simulink model "MSFartoystyring_2_CAC"  (R2018a)
settings: Solver=ode45  StartTime=tstart  StopTime=tstop  RelTol=1e-3  EnableMultiTasking=on
values from neighbouring files (symbols this model uses):
  c = 1    [run_2.m]    (also in run_task_1_4.m; run_task_1_6.m = 0; run_task_1_8_new.m)
  chi_t = atan2(WP(2,2)-WP(2,1),WP(1,2)-WP(1,1))    [run_2.m]
  dc_max = 25*(pi/180)    (= 0.436332312999)    [run_2.m]    (also in run_task_1_8_new.m)
  delta_e = 3*304.8    (= 914.4)    [run_2.m]
  delta_s = 3*304.8    (= 914.4)    [run_2.m]
  e_d = 2*304.8    (= 609.6)    [run_2.m]
  kappa = nc_max - U_t    (= 5.90117918517)    [run_2.m]
  kd_heading = 2*zeta*omegan*(m+km)-d    [run_2.m]    (also in run_task_1_8_new.m)
  kd_surge = 0    [run_2.m]
  ki_heading = omegan/10*kp_heading    [run_2.m]    (also in run_task_1_8_new.m)
  ki_surge = 0    [run_2.m]    (also in run_task_1_8_new.m = lambda^2)
  kp_heading = (m+km)*omegan^2-k    [run_2.m]    (also in run_task_1_8_new.m)
  kp_surge = 100    [run_2.m]    (also in run_task_1_8_new.m = 2*lambda)
  nc_max = (85/60)*2*pi    (= 8.90117918517)    [run_2.m]    (also in run_task_1_8_new.m)
  p0 = [1000 700]'    [run_2.m]    (also in run_task_1_4.m = zeros(2,1); run_task_1_6.m = zeros(2,1); run_task_1_8_new.m = zeros(2,1))
  psi0 = 60*pi/180    (= 1.0471975512)    [run_2.m]    (also in run_task_1_4.m = 0; run_task_1_6.m = 0; run_task_1_8_new.m = 0)
  r0 = 0    [run_2.m]    (also in run_task_1_4.m; run_task_1_6.m; run_task_1_8_new.m)
  s_d = 1*304.8    (= 304.8)    [run_2.m]
  tsamp = 10    [run_2.m]    (also in run_task_1_4.m; run_task_1_6.m; run_task_1_8_new.m)
  U_t = 3    [run_2.m]
  v0 = [6.63 0]'    [run_2.m]    (also in run_task_1_4.m; run_task_1_6.m = [0.001 0]'; run_task_1_8_new.m = [3 0]')
undefined symbols (not defined in the file or in its folder): msfartoystyring
settings Model: ExtModeAutoUpdateStatusClock=off  Creator=christh  LastModifiedBy=Anders Vagle
settings SolverCC: ZeroCrossAlgorithm=Adaptive
settings DataIOCC: LimitDataPoints=on  SaveFormat=Array
settings OptimizationCC: ExpressionDepthLimit=2147483647  InitFltsAndDblsToZero=on  LifeSpan=inf
settings DebuggingCC: UnderspecifiedInitializationDetection=Classic  MergeDetectMultiDrivingBlocksExec=none  MaxConsecutiveZCsMsg=none  SolverPrmCheckMsg=warning  FcnCallInpInsideContextMsg=warning  StateNameClashWarn=warning  SFUnexpectedBacktrackingDiag=warning  SFNoUnconditionalDefaultTransitionDiag=warning  SFExecutionAtInitializationDiag=none
settings HardwareCC: ProdBitPerPointer=32  ProdBitPerSizeT=32  ProdBitPerPtrDiffT=32  ProdLargestAtomicFloat=None  ProdIntDivRoundTo=Undefined  ProdEndianess=Unspecified  ProdWordSize=32  ProdHWDeviceType=32-bit Generic
settings ModelReferenceCC: PropagateSignalLabelsOutOfModel=off
settings CodeAppCC: StateflowObjectComments=on
settings GRTTargetCC: TargetLangStandard=C89/C90 (ANSI)  GeneratePreprocessorConditionals=Disable all  CombineOutputUpdateFcns=off  GRTInterface=on
settings ConfigComp: CovMetricSettings=dw  CovHtmlReporting=on  CovSaveCumulativeToWorkspaceVar=on  CovSaveSingleToWorkspaceVar=on  CovExternalEMLEnable=off

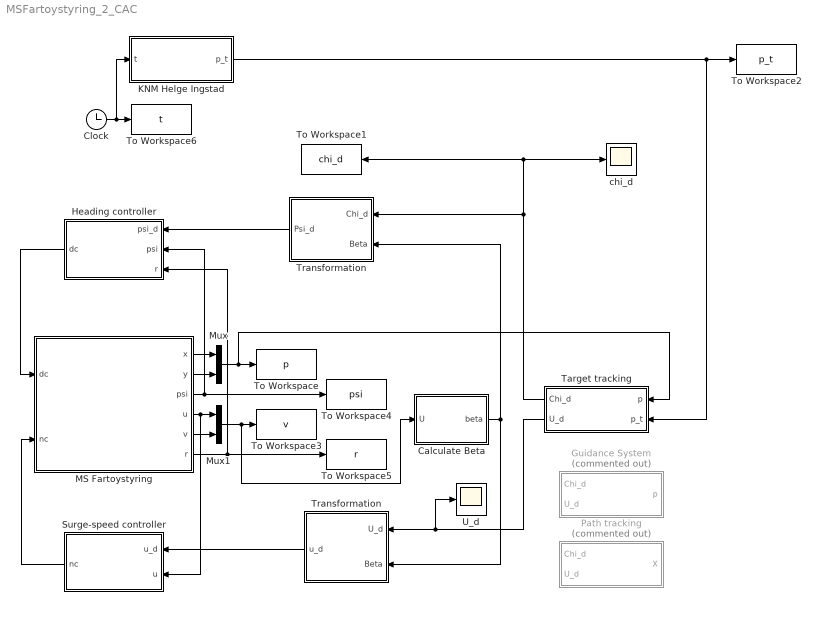
== system MSFartoystyring_2_CAC ==
  Calculate Beta : MATLAB Function  TreatAsAtomicUnit=on
  Clock : Clock
  Guidance System : Subsystem  Commented=on
  Heading controller : Subsystem
  KNM Helge Ingstad : Subsystem
  MS Fartoystyring : Subsystem  mask(MS Fartoystyring for Assignment 3 G&C){x0=p0(1), y0=p0(2), u0=v0(1), v0=v0(2), psi0=psi0, r0=r0, c=c}
      mask prompts: x0 "x(t0) (m)"; y0 "y(t0) (m)"; u0 "u(t0) (m/s)"; v0 "v(t0) (m/s)"; psi0 "psi(t0) (rad)"; r0 "r(t0) (rad/s)"; c "current (0 or 1)"
      mask help:
      | Block corresponding to Figure 1 in the assignment text. Gives the response of the ship.
      |
      | The design speed of MS Fartoystyring is u=8.23 m/s.
      |
      | Input:
      | dc: commanded rudder (rad), dmax=25*pi/180
      | nc: commanded shaft speed (rad/s), nmax=85*2*pi/60
      |
      | Output:
      | x: north pos (m)
      | y: east pos (m)
      | u: surge (m/s)
      | v: sway (m/s)
      | psi: heading (rad)
      | r: yaw (rad/s)
      mask Help: Comments, bugs and help requests can be directed to the TA. Email on course website.
  Mux : Mux  Inputs=2
  Mux1 : Mux  Inputs=2
  Path tracking : Subsystem  Commented=on
  Surge-speed controller : Subsystem
  Target tracking : Subsystem
  To Workspace : ToWorkspace  VariableName=p  SampleTime=tsamp
  To Workspace1 : ToWorkspace  VariableName=chi_d  SampleTime=tsamp
  To Workspace2 : ToWorkspace  VariableName=p_t  SampleTime=tsamp
  To Workspace3 : ToWorkspace  VariableName=v  SampleTime=tsamp
  To Workspace4 : ToWorkspace  VariableName=psi  SampleTime=tsamp
  To Workspace5 : ToWorkspace  VariableName=r  SampleTime=tsamp
  To Workspace6 : ToWorkspace  VariableName=t  SampleTime=tsamp
  Transformation : Subsystem
  "Transformation " : Subsystem
  U_d : Scope
  chi_d : Scope
  wires:
  Clock/1 -> KNM Helge Ingstad/1(t), To Workspace6/1
  MS Fartoystyring/1(x) -> Mux/1
  MS Fartoystyring/2(y) -> Mux/2
  MS Fartoystyring/4(u) -> Surge-speed controller/2("u "), Mux1/1
  MS Fartoystyring/5(v) -> Mux1/2
  Mux/1 -> Target tracking/1(p), To Workspace/1
  Mux1/1 -> Calculate Beta/1(U), To Workspace3/1
  MS Fartoystyring/6(r) -> Heading controller/3("r "), To Workspace5/1
  MS Fartoystyring/3(psi) -> Heading controller/2("psi "), To Workspace4/1
  Heading controller/1("dc ") -> MS Fartoystyring/1(dc)
  Surge-speed controller/1("nc ") -> MS Fartoystyring/2(nc)
  Transformation/1(Psi_d) -> Heading controller/1(psi_d)
  "Transformation "/1(u_d) -> Surge-speed controller/1(u_d)
  Calculate Beta/1(beta) -> Transformation/2(Beta), "Transformation "/2(Beta)
  Target tracking/1(Chi_d) -> chi_d/1, To Workspace1/1, Transformation/1(Chi_d)
  Target tracking/2(U_d) -> U_d/1, "Transformation "/1(U_d)
  KNM Helge Ingstad/1(p_t) -> To Workspace2/1, Target tracking/2(p_t)

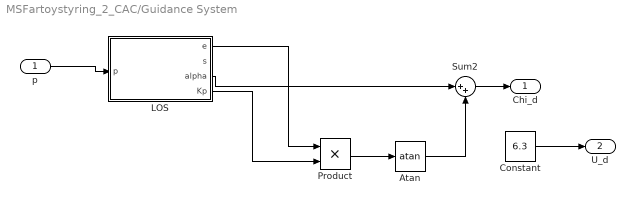
== system MSFartoystyring_2_CAC/Guidance System ==
  p : Inport
  Atan : Trigonometry  Operator=atan
  Constant : Constant  Value=6.3
  "LOS " : MATLAB Function  TreatAsAtomicUnit=on
  Product : Product
  Sum2 : Sum  Inputs=|++
  Chi_d : Outport
  U_d : Outport  Port=2
  wires:
  Constant/1 -> U_d/1
  "LOS "/3(alpha) -> Sum2/1
  Product/1 -> Atan/1
  "LOS "/4(Kp) -> Product/2
  "LOS "/1(e) -> Product/1
  Atan/1 -> Sum2/2
  Sum2/1 -> Chi_d/1
  p/1 -> "LOS "/1(p)

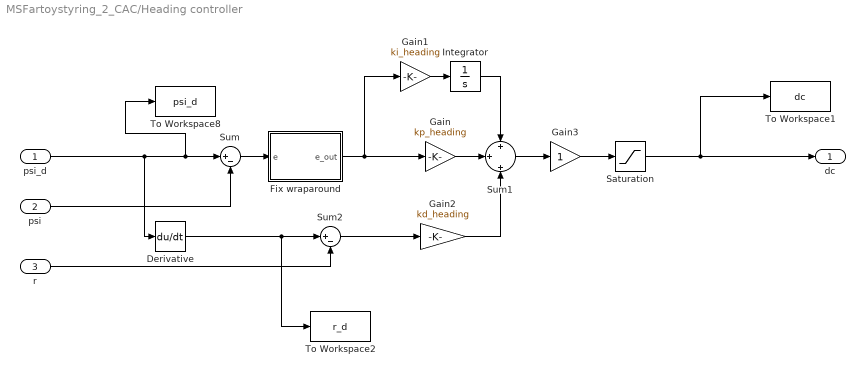
== system MSFartoystyring_2_CAC/Heading controller ==
  psi_d : Inport
  "psi " : Inport  Port=2
  "r " : Inport  Port=3
  Derivative : Derivative
  Fix wraparound : MATLAB Function  TreatAsAtomicUnit=on
  Gain : Gain  Gain=kp_heading
  Gain1 : Gain  Gain=ki_heading
  Gain2 : Gain  Gain=kd_heading
  Gain3 : Gain
  Integrator : Integrator
  Saturation : Saturate  UpperLimit=dc_max  LowerLimit=-dc_max
  Sum : Sum  Inputs=|+-
  Sum1 : Sum  Inputs=+|+|+
  Sum2 : Sum  Inputs=|+-
  To Workspace1 : ToWorkspace  VariableName=dc  SampleTime=tsamp
  To Workspace2 : ToWorkspace  VariableName=r_d  SampleTime=tsamp
  To Workspace8 : ToWorkspace  VariableName=psi_d  SampleTime=tsamp
  "dc " : Outport
  wires:
  Sum/1 -> Fix wraparound/1(e)
  Gain1/1 -> Integrator/1
  Sum1/1 -> Gain3/1
  Gain/1 -> Sum1/2
  Gain2/1 -> Sum1/3
  Gain3/1 -> Saturation/1
  Integrator/1 -> Sum1/1
  "psi "/1 -> Sum/2
  Derivative/1 -> To Workspace2/1, Sum2/1
  psi_d/1 -> To Workspace8/1, Sum/1, Derivative/1
  Sum2/1 -> Gain2/1
  "r "/1 -> Sum2/2
  Saturation/1 -> To Workspace1/1, "dc "/1
  Fix wraparound/1(e_out) -> Gain/1, Gain1/1

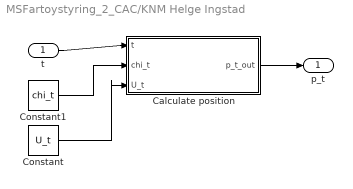
== system MSFartoystyring_2_CAC/KNM Helge Ingstad ==
  t : Inport
  Calculate position : MATLAB Function  TreatAsAtomicUnit=on
  Constant : Constant  Value=U_t
  Constant1 : Constant  Value=chi_t
  p_t : Outport
  wires:
  t/1 -> Calculate position/1(t)
  Calculate position/1(p_t_out) -> p_t/1
  Constant1/1 -> Calculate position/2(chi_t)
  Constant/1 -> Calculate position/3(U_t)

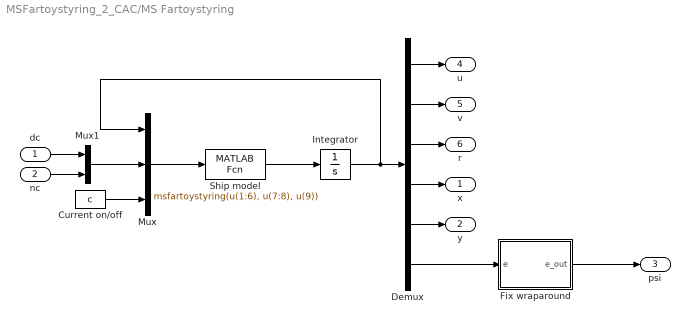
== system MSFartoystyring_2_CAC/MS Fartoystyring ==
  dc : Inport
  nc : Inport  Port=2
  Current on/off : Constant  Value=c
  Demux : Demux  Outputs=6
  Fix wraparound : MATLAB Function  TreatAsAtomicUnit=on
  Integrator : Integrator  InitialCondition=[u0 v0 r0 x0 y0 psi0]'
  Mux : Mux  Inputs=3
  Mux1 : Mux  Inputs=2
  Ship model : MATLABFcn  MATLABFcn=msfartoystyring(u(1:6), u(7:8), u(9))  OutputDimensions=6
  x : Outport
  y : Outport  Port=2
  psi : Outport  Port=3
  u : Outport  Port=4
  v : Outport  Port=5
  r : Outport  Port=6
  wires:
  Integrator/1 -> Mux/1, Demux/1
  Mux1/1 -> Mux/2
  dc/1 -> Mux1/1
  nc/1 -> Mux1/2
  Demux/1 -> u/1
  Demux/2 -> v/1
  Demux/3 -> r/1
  Demux/4 -> x/1
  Demux/5 -> y/1
  Current on/off/1 -> Mux/3
  Ship model/1 -> Integrator/1
  Mux/1 -> Ship model/1
  Fix wraparound/1(e_out) -> psi/1
  Demux/6 -> Fix wraparound/1(e)

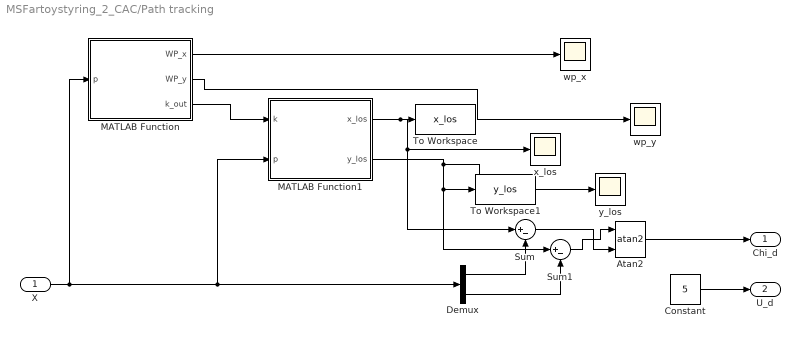
== system MSFartoystyring_2_CAC/Path tracking ==
  X : Inport
  Atan2 : Trigonometry  Operator=atan2
  Constant : Constant  Value=5
  Demux : Demux  Outputs=2
  MATLAB Function : MATLAB Function  TreatAsAtomicUnit=on
  MATLAB Function1 : MATLAB Function  TreatAsAtomicUnit=on
  Sum : Sum  Inputs=|+-
  Sum1 : Sum  Inputs=|+-
  To Workspace : ToWorkspace  VariableName=x_los  SampleTime=-1
  To Workspace1 : ToWorkspace  VariableName=y_los  SampleTime=-1
  wp_x : Scope
  wp_y : Scope
  x_los : Scope
  y_los : Scope
  Chi_d : Outport
  U_d : Outport  Port=2
  wires:
  Constant/1 -> U_d/1
  X/1 -> MATLAB Function/1(p), MATLAB Function1/2(p), Demux/1
  Demux/1 -> Sum/2
  Demux/2 -> Sum1/2
  Atan2/1 -> Chi_d/1
  MATLAB Function/1(WP_x) -> wp_x/1
  MATLAB Function/2(WP_y) -> wp_y/1
  MATLAB Function/3(k_out) -> MATLAB Function1/1(k)
  MATLAB Function1/2(y_los) -> y_los/1, Sum1/1, To Workspace1/1
  MATLAB Function1/1(x_los) -> x_los/1, Sum/1, To Workspace/1
  Sum/1 -> Atan2/2
  Sum1/1 -> Atan2/1

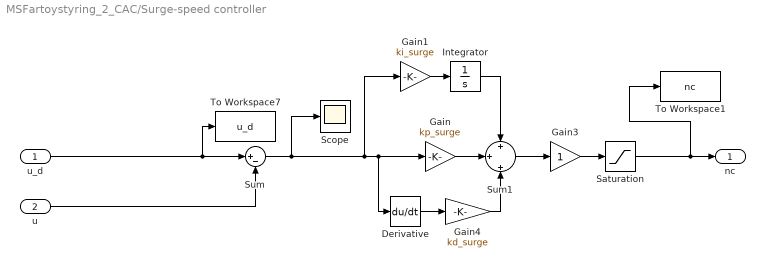
== system MSFartoystyring_2_CAC/Surge-speed controller ==
  u_d : Inport
  "u " : Inport  Port=2
  Derivative : Derivative
  Gain : Gain  Gain=kp_surge
  Gain1 : Gain  Gain=ki_surge
  Gain3 : Gain
  Gain4 : Gain  Gain=kd_surge
  Integrator : Integrator
  Saturation : Saturate  UpperLimit=nc_max  LowerLimit=0
  Scope : Scope
  Sum : Sum  Inputs=|+-
  Sum1 : Sum  Inputs=+|+|+
  To Workspace1 : ToWorkspace  VariableName=nc  SampleTime=tsamp
  To Workspace7 : ToWorkspace  VariableName=u_d  SampleTime=tsamp
  "nc " : Outport
  wires:
  Gain1/1 -> Integrator/1
  Sum1/1 -> Gain3/1
  Gain/1 -> Sum1/2
  u_d/1 -> To Workspace7/1, Sum/1
  Gain3/1 -> Saturation/1
  Integrator/1 -> Sum1/1
  "u "/1 -> Sum/2
  Sum/1 -> Scope/1, Derivative/1, Gain/1, Gain1/1
  Derivative/1 -> Gain4/1
  Gain4/1 -> Sum1/3
  Saturation/1 -> To Workspace1/1, "nc "/1

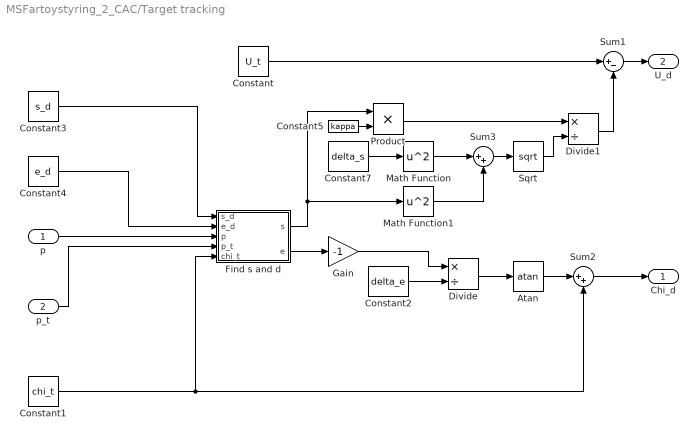
== system MSFartoystyring_2_CAC/Target tracking ==
  p : Inport
  p_t : Inport  Port=2
  Atan : Trigonometry  Operator=atan
  Constant : Constant  Value=U_t
  Constant1 : Constant  Value=chi_t
  Constant2 : Constant  Value=delta_e
  Constant3 : Constant  Value=s_d
  Constant4 : Constant  Value=e_d
  Constant5 : Constant  Value=kappa
  Constant7 : Constant  Value=delta_s
  Divide : Product  Inputs=*/
  Divide1 : Product  Inputs=*/
  Find s and d : MATLAB Function  TreatAsAtomicUnit=on
  Gain : Gain  Gain=-1
  Math Function : Math  Operator=square  SaturateOnIntegerOverflow=on
  Math Function1 : Math  Operator=square  SaturateOnIntegerOverflow=on
  Product : Product
  Sqrt : Sqrt  SaturateOnIntegerOverflow=on
  Sum1 : Sum  Inputs=|+-
  Sum2 : Sum  Inputs=|++
  Sum3 : Sum  Inputs=|++
  Chi_d : Outport
  U_d : Outport  Port=2
  wires:
  p/1 -> Find s and d/3(p)
  Atan/1 -> Sum2/1
  Sum2/1 -> Chi_d/1
  Divide/1 -> Atan/1
  Constant2/1 -> Divide/2
  Find s and d/2(e) -> Gain/1
  Gain/1 -> Divide/1
  Constant3/1 -> Find s and d/1(s_d)
  Constant4/1 -> Find s and d/2(e_d)
  p_t/1 -> Find s and d/4(p_t)
  Sum1/1 -> U_d/1
  Constant/1 -> Sum1/1
  Find s and d/1(s) -> Math Function1/1, Product/1
  Constant5/1 -> Product/2
  Product/1 -> Divide1/1
  Sqrt/1 -> Divide1/2
  Constant7/1 -> Math Function/1
  Math Function/1 -> Sum3/1
  Math Function1/1 -> Sum3/2
  Sum3/1 -> Sqrt/1
  Divide1/1 -> Sum1/2
  Constant1/1 -> Sum2/2, Find s and d/5(chi_t)

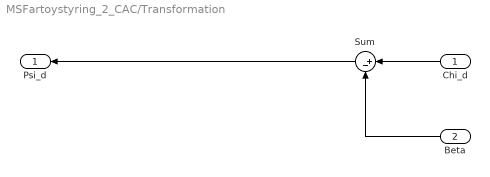
== system MSFartoystyring_2_CAC/Transformation ==
  Chi_d : Inport
  Beta : Inport  Port=2
  Sum : Sum  Inputs=|+-
  Psi_d : Outport
  wires:
  Sum/1 -> Psi_d/1
  Beta/1 -> Sum/2
  Chi_d/1 -> Sum/1

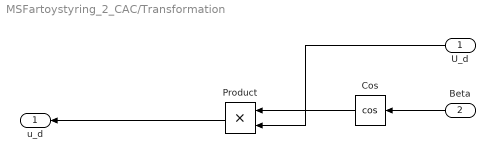
== system MSFartoystyring_2_CAC/Transformation  ==
  U_d : Inport
  Beta : Inport  Port=2
  Cos : Trigonometry  Operator=cos
  Product : Product
  u_d : Outport
  wires:
  Cos/1 -> Product/1
  U_d/1 -> Product/2
  Beta/1 -> Cos/1
  Product/1 -> u_d/1

== matlab function MSFartoystyring_2_CAC/Guidance System/LOS  ==
  settings: updateMethod=DISCRETE  sampleTime=tsamp
  data: p input; e output; s output; alpha output; Kp output
function [e,s,alpha, Kp] = fcn(p)
    persistent k;
    
    if isempty(k)
        k=1;
    end
    WP = [0 -3500 -7000 -12000 -15000 -18000;
          0 -2500 -500  -3500  -500   -2000];

    % Position
    x = p(1);
    y = p(2);
    
    x_k_1 = WP(1, k + 1);
    y_k_1 = WP(2, k + 1); 
    
    x_k = WP(1,k);
    y_k = WP(2,k);
    
    if (((x_k-x)^2+(y_k-y)^2)<=2*304.8)
        k = k + 1
    end
    
    alpha = atan2(y_k_1 - y_k, x_k_1 - x_k);
    R = [ cos(alpha) -sin(alpha) ; sin(alpha) cos(alpha) ];
    eps = R'*[(x - x_k) (y - y_k)]';
    e = eps(1);
    s = eps(2);
    delta = sqrt(R*R - e*e);
    Kp = -1/delta

end

== matlab function MSFartoystyring_2_CAC/Path tracking/MATLAB Function ==
  settings: updateMethod=DISCRETE  sampleTime=tsamp
  data: WP_x output; p input; WP_y output; k_out output
function [WP_x, WP_y, k_out] = active_waypoint(p)

persistent k
persistent t
if isempty(k)
   k = 1
end
if isempty(t)
    t = 1;
else 
    t = t + 1;
end

%WP = load('WP.mat') % aids

WP = [0 -3500 -7000 -12000 -15000 -18000;
      0 -2500 -500  -3500  -500   -2000];

x_k = WP(1,k);
y_k = WP(2,k);

x = p(1);
y = p(2);
%distance_to_waypoint = (x_k-x)^2+(y_k-y)^2
if (((x_k-x)^2+(y_k-y)^2)<=(2*304.8)^2 && k<6)
    k = k + 1
    t*10
end

WP_x = WP(1,k);
WP_y = WP(2,k);
k_out = k;

== matlab function MSFartoystyring_2_CAC/Path tracking/MATLAB Function1 ==
  settings: updateMethod=DISCRETE  sampleTime=tsamp
  data: k input; x_los output; p input; y_los output
function [x_los, y_los] = LOS_points(k, p)

WP = [0 -3500 -7000 -12000 -15000 -18000;
      0 -2500 -500  -3500  -500   -2000];
R = 5*304.8;

x = p(1);
y = p(2);

x_k = WP(1,k);
y_k = WP(2,k);

if k > 1
x_k_1 = WP(1,k-1); %x_k_1 = WP(1,k+1);
y_k_1 = WP(2,k-1); %y_k_1 = WP(2,k+1);
else
    x_k_1 = 1000;
    y_k_1 = 700;
end

delta_x = x_k - x_k_1; %delta_x = x_k_1 - x_k;
delta_y = y_k - y_k_1; %delta_y = y_k_1 - y_k;

d = delta_y / delta_x;

if (((x_k-x)^2+(y_k-y)^2)<=(R)^2)
    R = sqrt((x_k-x)^2+(y_k-y)^2);
end

if delta_x==0
    x_los = x_k_1;
    if delta_y > 0
        y_los = y + sqrt(R^2-(x_los-x)^2);
    else
        y_los = y - sqrt(R^2-(x_los-x)^2);
    end
else
    g = y_k_1 - d*x_k_1;
    
    a = 1 + d^2;
    b = 2*(d*g - d*y - x);
    c = x^2 + y^2 + g^2 - 2*g*y - R^2;
    
    if delta_x > 0
        %pos_delta_x = b^2 - 4*a*c
        x_los = (-b + sqrt(b^2 - 4*a*c))/(2*a);
    else
        %neg_delta_x = b^2 - 4*a*c
        x_los = (-b - sqrt(b^2 - 4*a*c))/(2*a);
    end
    
    y_los = d*(x_los - x_k_1) + y_k_1;
end

== matlab function MSFartoystyring_2_CAC/Heading controller/Fix wraparound ==
  data: e input; e_out output
function e_out = fix_wraparound(e)


e_out = mod(e+pi,2*pi)-pi;

% if e > pi
%     e_out = e - n*(2*pi);
% elseif e < -pi
%     e_out = e + n*(2*pi);
% else
%     e_out = e;
% end

== matlab function MSFartoystyring_2_CAC/MS Fartoystyring/Fix wraparound ==
  data: e input; e_out output
function e_out = fix_wraparound(e)


e_out = mod(e+pi,2*pi)-pi;

% if e > pi
%     e_out = e - n*(2*pi);
% elseif e < -pi
%     e_out = e + n*(2*pi);
% else
%     e_out = e;
% end

== matlab function MSFartoystyring_2_CAC/Calculate Beta ==
  data: U input; beta output
function beta = U_to_beta(U)
u = U(1);
v = U(2);
beta = asin(v/sqrt(u^2 +v^2));
end

== matlab function MSFartoystyring_2_CAC/KNM Helge Ingstad/Calculate position ==
  settings: updateMethod=DISCRETE  sampleTime=tsamp
  data: t input; p_t_out output; chi_t input; U_t input
function p_t_out = helgeingstad(t, chi_t, U_t)
% Calculate position of ship to be tracked

persistent p_t
if isempty(p_t)
    p_t = [-3500, -2500]'; % North, East
end

x_t = p_t(1);
y_t = p_t(2);

WP = [0 -3500 -7000 -12000 -15000 -18000;
      0 -2500 -500  -3500  -500   -2000];

y_t = WP(2,2)+U_t*sin(chi_t)*t;
x_t = WP(1,2)+U_t*cos(chi_t)*t;

% x_t_dot = U_t*sin(chi_t);
% y_t_dot = U_t*cos(chi_t);
% 
% x_t = x_t + x_t_dot*t;
% y_t = y_t + y_t_dot*t;


p_t_out = [x_t, y_t]';

== matlab function MSFartoystyring_2_CAC/Target tracking/Find s and d ==
  data: s_d input; s output; e_d input; p input; p_t input; chi_t input; e output
function [s, e] = fcn(s_d, e_d, p, p_t, chi_t)

chi_t = sin(chi_t);

R = [cos(chi_t) -sin(chi_t);
     sin(chi_t) cos(chi_t)];
 
s = s_d + R*(p - p_t);
e = e_d + R*(p - p_t);
